simulink model "ParachuteSimV1"  (R2024b)
settings: Solver=ode5  StartTime=0.0  StopTime=1000  FixedStep=.1  RelTol=1e-3
model workspace (MAT data in the model file):
  dayOfYear = 182
  drogueArea = 1.2
  drogueCd = 2.2
  mass = 45
  rocketHorizontalArea = 3.2
  rocketHorizontalCd = 0.8
  rocketHorizontalCd1 = 0.4
  rocketMass = 165
  secOfDayUTC = 43200
  test = 1
  year = 2025
values from neighbouring files (symbols this model uses):
  apogeeHeight = ZeDeviation.*randn(numSim,1) + ZeInitial    [ParachuteSimV1.m]
  density = 0.004    [SnatchForceCalc.m]    (also in SnatchForceCalcTR.m = 1.2)
  eastwardVelocity = 30    [ParachuteSimV1.m]
  g = 9.81    [ParachuteSimV1.m]
  lattitude = 40.861903    [ParachuteSimV1.m]
  longitude = -119.113646    [ParachuteSimV1.m]
  northwardVelocity = 30    [ParachuteSimV1.m]
undefined symbols (not defined in the file or in its folder): DiscIntNeverNeededParam, Earth, WGS84, WInitialMPS
libraries: simulink x5, aerolibatmos2 x1, aerolibtransform2 x1
settings Model: PacingRate=0.100000  Creator=siyfo  LastModifiedBy=siyfo

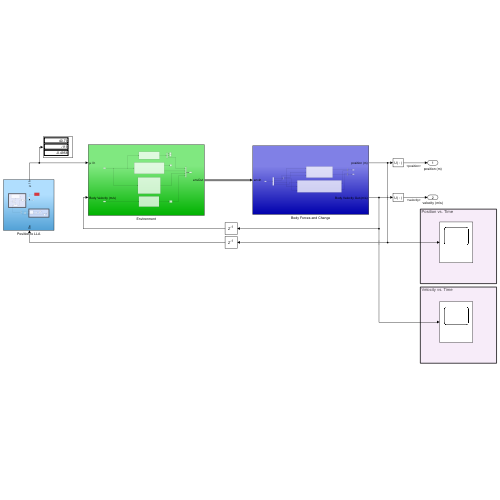
[thumbnail: Simulink's stored preview of the top-level diagram]
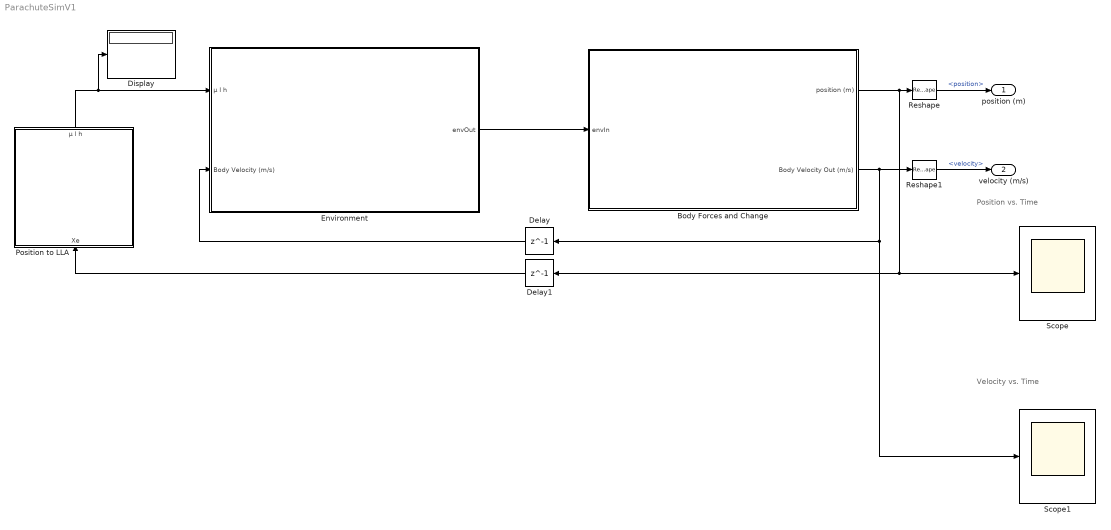
== system ParachuteSimV1 ==
  note: Position vs. Time
  note: Velocity vs. Time
  Body Forces and Change : Subsystem
  Delay : Delay  DelayLength=1  InitialCondition=0
  Delay1 : Delay  DelayLength=1  InitialCondition=0
  Display : Display
  Environment : Subsystem
  Position to LLA : Subsystem
      settings: PortSchema="{\"entries\":[{\"content\":{\"sides\":[{\"content\":{},\"type\":\"ConnectorPlacement.EquallySpacedRectSide\",\"uuid\":\"395108a1-2b9e-4f25-b149-7e7a55081f25\"},{\"content\":{\"side\":\"RIGHT\"},\"type\":\"ConnectorPlacement.EquallySpacedRectSide\",\"uuid\":\"27b5f7e2-b846-4579-8541-6937c01c751e\"},{\"content\":{\"connectorIds\":[\"Out1\"],\"side\":\"TOP\"},\"type\":\"ConnectorPlacement.EquallySpacedRectSide\",\"uuid\":\"43ca551c-6ed4-44f9-86d9-aa9f5a015e71\"},{\"content\":{\"connectorIds\":[\"In1\"],\"side\":\"BOTTOM\"},\"type\":\"ConnectorPlacement.EquallySpacedRectSide\",\"uuid\":\"6a16c409-2c2d-4a86-9d37-b69d0f58a179\"}]},\"type\":\"ConnectorPlacement.EquallySpacedConnector\",\"uuid\":\"59df7613-7675-4f40-93a5-9c85f63bdba2\"}],\"packageUris\":[\"http://schema.mathworks.com/mf0/Connector/R2020b\"],\"version\":\"1.0\"}"
  Reshape : Reshape  OutputDimensions=[1]
  Reshape1 : Reshape  OutputDimensions=[1]
  Scope : Scope
  Scope1 : Scope
  position (m) : Outport
  velocity (m/s) : Outport  Port=2  Unit=m/s
  wires:
  Environment/1(envOut) -> Body Forces and Change/1(envIn)
  Body Forces and Change/2(Body Velocity Out (m/s)) -> Reshape1/1, Delay/1, Scope1/1
  Position to LLA/1(μ l h) -> Display/1, Environment/1(μ l h)
  Delay1/1 -> Position to LLA/1(Xe)
  Delay/1 -> Environment/2(Body Velocity (m/s))
  Body Forces and Change/1(position (m)) -> Reshape/1, Scope/1, Delay1/1
  Reshape/1 -> position (m)/1  "<position>"
  Reshape1/1 -> velocity (m/s)/1  "<velocity>"

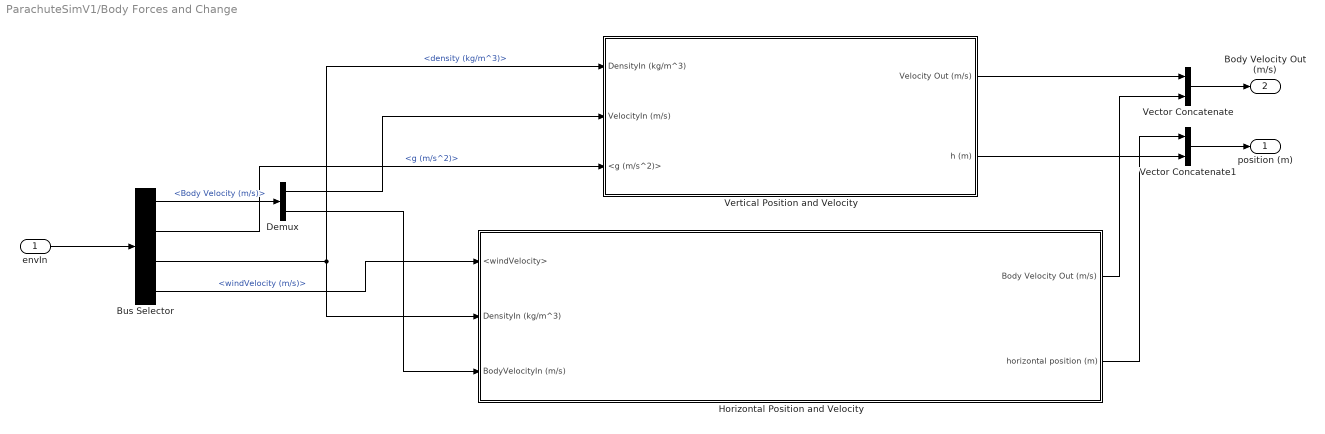
== system ParachuteSimV1/Body Forces and Change ==
  envIn : Inport
  Bus Selector : BusSelector  OutputSignals=Body Velocity (m/s),g (m/s^2),density (kg/m^3),windVelocity (m/s)
  Demux : Demux  Outputs=2
  Horizontal Position and Velocity : Subsystem
  Vector Concatenate : Concatenate  Mode=Multidimensional array
  Vector Concatenate1 : Concatenate  Mode=Multidimensional array
  Vertical Position and Velocity : Subsystem
  position (m) : Outport
  Body Velocity Out (m/s) : Outport  Port=2
  wires:
  envIn/1 -> Bus Selector/1
  Bus Selector/1 -> Demux/1  "<Body Velocity (m/s)>"
  Bus Selector/4 -> Horizontal Position and Velocity/1(<windVelocity>)  "<windVelocity (m/s)>"
  Bus Selector/3 -> Vertical Position and Velocity/1(DensityIn (kg/m^3)), Horizontal Position and Velocity/2(DensityIn (kg/m^3))  "<density (kg/m^3)>"
  Bus Selector/2 -> Vertical Position and Velocity/3(<g (m/s^2)>)  "<g (m/s^2)>"
  Vertical Position and Velocity/1(Velocity Out (m/s)) -> Vector Concatenate/1
  Demux/2 -> Horizontal Position and Velocity/3(BodyVelocityIn (m/s))
  Demux/1 -> Vertical Position and Velocity/2(VelocityIn (m/s))
  Vertical Position and Velocity/2(h (m)) -> Vector Concatenate1/2
  Vector Concatenate/1 -> Body Velocity Out (m/s)/1
  Vector Concatenate1/1 -> position (m)/1
  Horizontal Position and Velocity/2(horizontal position (m)) -> Vector Concatenate1/1
  Horizontal Position and Velocity/1(Body Velocity Out (m/s)) -> Vector Concatenate/2

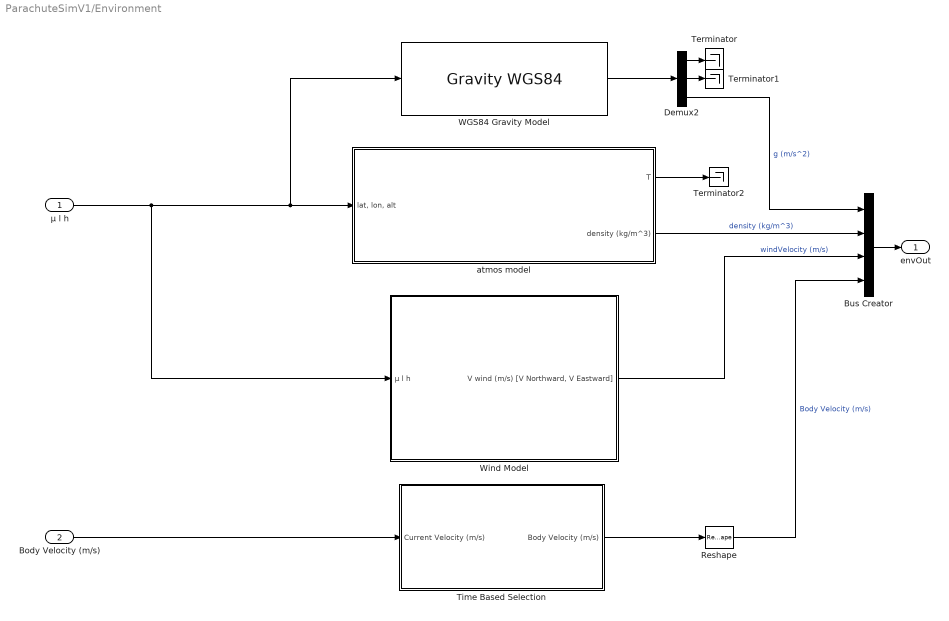
== system ParachuteSimV1/Environment ==
  μ l h : Inport
  Body Velocity (m/s) : Inport  Port=2
  Bus Creator : BusCreator  Inputs=g (m/s^2),density (kg/m^3),windVelocity (m/s),Body Velocity (m/s)
  Demux2 : Demux  Outputs=3
  Reshape : Reshape
  Terminator : Terminator
  Terminator1 : Terminator
  Terminator2 : Terminator
  Time Based Selection : Subsystem
  "WGS84 Gravity Model  " : GravityWGS84
  Wind Model : Subsystem
  atmos model : Subsystem
  envOut : Outport
  wires:
  atmos model/1(T) -> Terminator2/1
  Demux2/1 -> Terminator/1
  Demux2/2 -> Terminator1/1
  Demux2/3 -> Bus Creator/1  "g (m/s^2)"
  "WGS84 Gravity Model  "/1 -> Demux2/1
  atmos model/2(density (kg/m^3)) -> Bus Creator/2  "density (kg/m^3)"
  μ l h/1 -> atmos model/1("lat, lon, alt"), "WGS84 Gravity Model  "/1, Wind Model/1(μ l h)
  Wind Model/1("V wind (m/s) [V Northward, V Eastward]") -> Bus Creator/3  "windVelocity (m/s)"
  Bus Creator/1 -> envOut/1
  Body Velocity (m/s)/1 -> Time Based Selection/1(Current Velocity (m/s))
  Time Based Selection/1(Body Velocity (m/s)) -> Reshape/1
  Reshape/1 -> Bus Creator/4  "Body Velocity (m/s)"

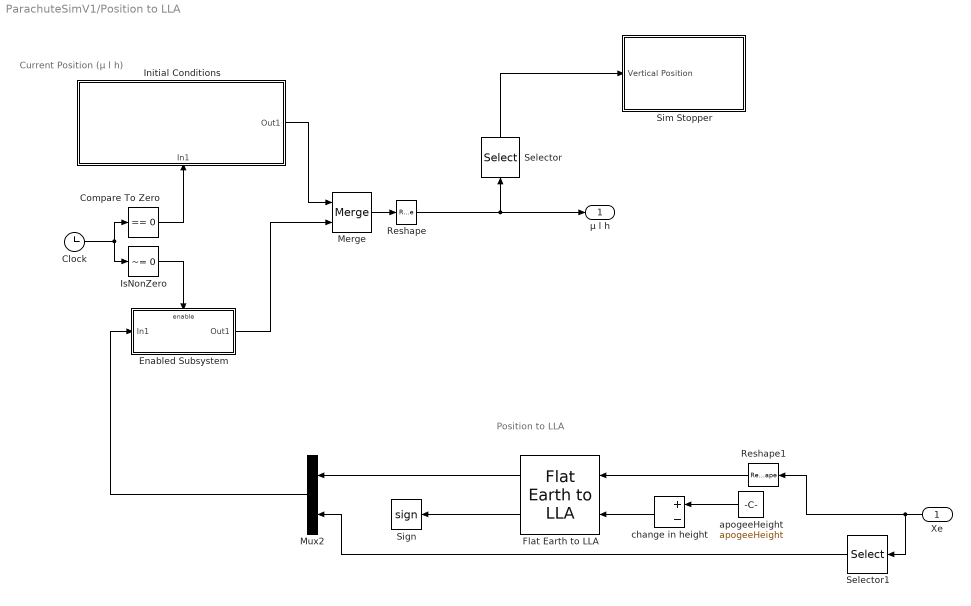
== system ParachuteSimV1/Position to LLA ==
  note: Position to LLA
  note: Current Position (μ l h)
  Xe : Inport
  Clock : Clock
  Compare To Zero : simulink/Logic and Bit Operations/Compare To Zero  relop===  OutDataTypeStr=uint8
  Enabled Subsystem : Subsystem  TreatAsAtomicUnit=on
  Flat Earth to LLA : aerolibtransform2/Flat Earth to LLA  units=Metric (MKS)  ptype=Earth (WGS84)  F=1/298.257223563  R=6378137  refPosPort=off  LL0=[lattitude longitude]  psi=90
  Initial Conditions : Subsystem
      settings: PortSchema="{\"entries\":[{\"content\":{\"sides\":[{\"content\":{},\"type\":\"ConnectorPlacement.EquallySpacedRectSide\",\"uuid\":\"693e8934-6ee4-461b-8cf6-42b2b2261af3\"},{\"content\":{\"connectorIds\":[\"Out1\"],\"side\":\"RIGHT\"},\"type\":\"ConnectorPlacement.EquallySpacedRectSide\",\"uuid\":\"27a2a18d-addc-401c-ab89-c55f8d21a6b0\"},{\"content\":{\"side\":\"TOP\"},\"type\":\"ConnectorPlacement.EquallySpacedRectSide\",\"uuid\":\"aace6f03-20fd-4ea0-8b41-e6402498191a\"},{\"content\":{\"connectorIds\":[\"In1\"],\"side\":\"BOTTOM\"},\"type\":\"ConnectorPlacement.EquallySpacedRectSide\",\"uuid\":\"e2c8b452-2239-4d25-8a3f-abbb82eaafca\"}]},\"type\":\"ConnectorPlacement.EquallySpacedConnector\",\"uuid\":\"08404bb2-7ad5-42d3-9682-7974a009b565\"}],\"packageUris\":[\"http://schema.mathworks.com/mf0/Connector/R2020b\"],\"version\":\"1.0\"}"
  IsNonZero : simulink/Logic and Bit Operations/Compare To Zero  relop=~=  OutDataTypeStr=boolean
      settings: LibrarySourceBlock=|
      | simulink/Quick Insert/Logic and Bit
      | Operations/IsNonZero
  Merge : Merge
  Mux2 : Mux  Inputs=2
  Reshape : Reshape
  Reshape1 : Reshape
  Selector : Selector  InputPortWidth=3  IndexOptions=Index vector (dialog)  Indices=[3]  OutputSizes=1
  Selector1 : Selector  InputPortWidth=3  IndexOptions=Index vector (dialog)  Indices=[3]  OutputSizes=1
  Sign : Signum
  Sim Stopper : Subsystem
  apogeeHeight : Constant  Value=apogeeHeight
  change in height : Sum  Inputs=+-
  μ l h : Outport
  wires:
  IsNonZero/1 -> Enabled Subsystem/Enable
  Compare To Zero/1 -> Initial Conditions/1(In1)
  Initial Conditions/1(Out1) -> Merge/1
  Enabled Subsystem/1(Out1) -> Merge/2
  Flat Earth to LLA/1 -> Mux2/1
  Clock/1 -> Compare To Zero/1, IsNonZero/1
  Merge/1 -> Reshape/1
  Xe/1 -> Reshape1/1, Selector1/1
  Flat Earth to LLA/2 -> Sign/1
  Selector1/1 -> Mux2/2
  apogeeHeight/1 -> change in height/1
  change in height/1 -> Flat Earth to LLA/2
  Reshape1/1 -> Flat Earth to LLA/1
  Mux2/1 -> Enabled Subsystem/1(In1)
  Selector/1 -> Sim Stopper/1(Vertical Position)
  Reshape/1 -> Selector/1, μ l h/1

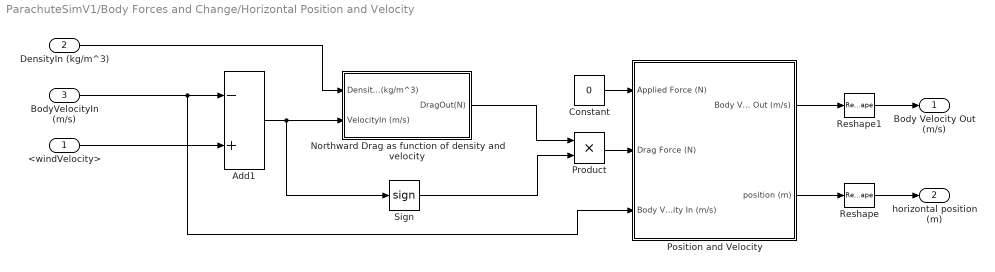
== system ParachuteSimV1/Body Forces and Change/Horizontal Position and Velocity ==
  <windVelocity> : Inport
  DensityIn (kg/m^3) : Inport  Port=2
  BodyVelocityIn (m/s) : Inport  Port=3
  Add1 : Sum  Inputs=-+
  Constant : Constant  Value=0
  Northward Drag as function of density and velocity : Subsystem
  Position and Velocity : Subsystem
  Product : Product
  Reshape : Reshape
  Reshape1 : Reshape
  Sign : Signum
  Body Velocity Out (m/s) : Outport
  horizontal position (m) : Outport  Port=2  OutDataTypeStr=fixdt('double', 'DataTypeOverride', 'Off')
  wires:
  <windVelocity>/1 -> Add1/2
  Constant/1 -> Position and Velocity/1(Applied Force (N))
  Sign/1 -> Product/2
  DensityIn (kg/m^3)/1 -> Northward Drag as function of density and velocity/1(DensityIn (kg/m^3))
  Position and Velocity/2(position (m)) -> Reshape/1
  Add1/1 -> Sign/1, Northward Drag as function of density and velocity/2(VelocityIn (m/s))
  Position and Velocity/1(Body Velocity Out (m/s)) -> Reshape1/1
  BodyVelocityIn (m/s)/1 -> Position and Velocity/3(Body Velocity In (m/s)), Add1/1
  Reshape/1 -> horizontal position (m)/1
  Reshape1/1 -> Body Velocity Out (m/s)/1
  Northward Drag as function of density and velocity/1(DragOut(N)) -> Product/1
  Product/1 -> Position and Velocity/2(Drag Force (N))

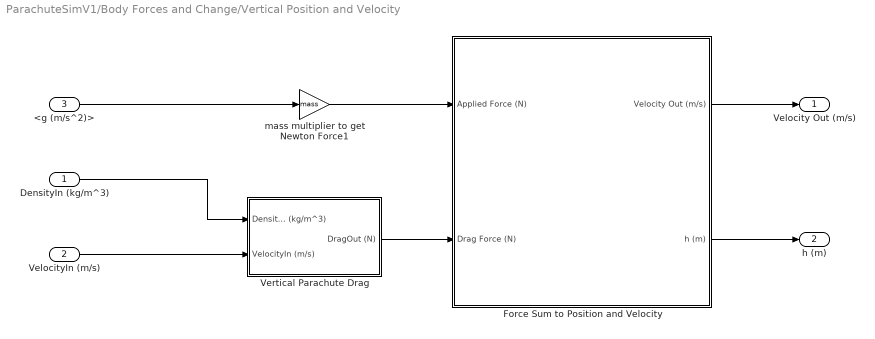
== system ParachuteSimV1/Body Forces and Change/Vertical Position and Velocity ==
  DensityIn (kg/m^3) : Inport
  VelocityIn (m/s) : Inport  Port=2
  <g (m/s^2)> : Inport  Port=3
  Force Sum to Position and Velocity : Subsystem
  Vertical Parachute Drag : Subsystem
  mass multiplier to get Newton Force1 : Gain  Gain=mass
  Velocity Out (m/s) : Outport
  h (m) : Outport  Port=2
  wires:
  Vertical Parachute Drag/1(DragOut (N)) -> Force Sum to Position and Velocity/2(Drag Force (N))
  DensityIn (kg/m^3)/1 -> Vertical Parachute Drag/1(DensityIn (kg/m^3))
  VelocityIn (m/s)/1 -> Vertical Parachute Drag/2(VelocityIn (m/s))
  mass multiplier to get Newton Force1/1 -> Force Sum to Position and Velocity/1(Applied Force (N))
  <g (m/s^2)>/1 -> mass multiplier to get Newton Force1/1
  Force Sum to Position and Velocity/2(h (m)) -> h (m)/1
  Force Sum to Position and Velocity/1(Velocity Out (m/s)) -> Velocity Out (m/s)/1

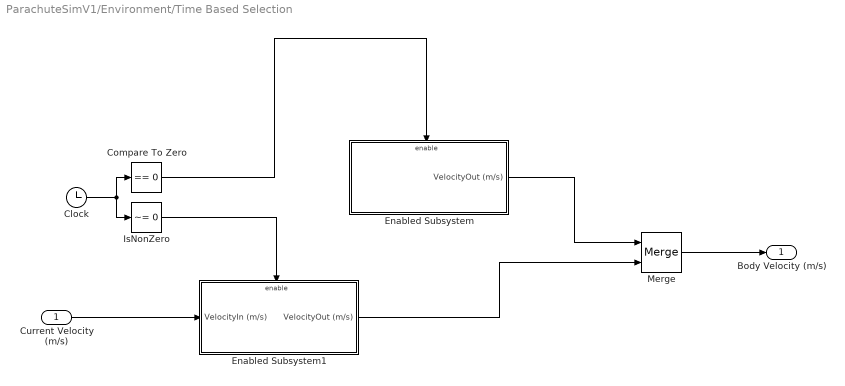
== system ParachuteSimV1/Environment/Time Based Selection ==
  Current Velocity (m/s) : Inport
  Clock : Clock
  Compare To Zero : simulink/Logic and Bit Operations/Compare To Zero  relop===  OutDataTypeStr=uint8
  Enabled Subsystem : Subsystem  TreatAsAtomicUnit=on
  Enabled Subsystem1 : Subsystem  TreatAsAtomicUnit=on
  IsNonZero : simulink/Logic and Bit Operations/Compare To Zero  relop=~=  OutDataTypeStr=boolean
  Merge : Merge
  Body Velocity (m/s) : Outport
  wires:
  Current Velocity (m/s)/1 -> Enabled Subsystem1/1(VelocityIn (m/s))
  Clock/1 -> Compare To Zero/1, IsNonZero/1
  IsNonZero/1 -> Enabled Subsystem1/Enable
  Compare To Zero/1 -> Enabled Subsystem/Enable
  Enabled Subsystem1/1(VelocityOut (m/s)) -> Merge/2
  Enabled Subsystem/1(VelocityOut (m/s)) -> Merge/1
  Merge/1 -> Body Velocity (m/s)/1

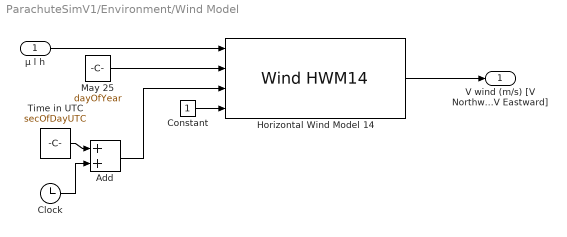
== system ParachuteSimV1/Environment/Wind Model ==
  μ l h : Inport
  Add : Sum
  Clock : Clock
  Constant : Constant
  Horizontal Wind Model 14 : WindHWM14  model=Total  action=Warning
  May 25 : Constant  Value=dayOfYear
  Time in UTC : Constant  Value=secOfDayUTC
  "V wind (m/s) [V Northward, V Eastward]" : Outport
  wires:
  May 25/1 -> Horizontal Wind Model 14/2
  Add/1 -> Horizontal Wind Model 14/3
  Time in UTC/1 -> Add/1
  Constant/1 -> Horizontal Wind Model 14/4
  Clock/1 -> Add/2
  μ l h/1 -> Horizontal Wind Model 14/1
  Horizontal Wind Model 14/1 -> "V wind (m/s) [V Northward, V Eastward]"/1

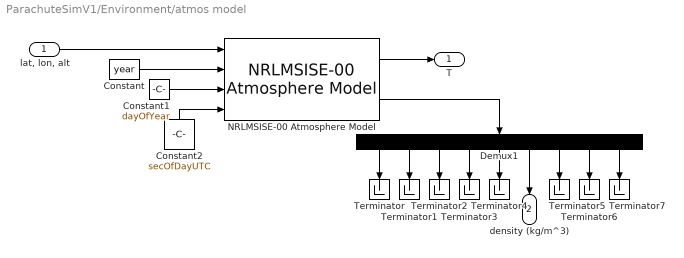
== system ParachuteSimV1/Environment/atmos model ==
  "lat, lon, alt" : Inport
  Constant : Constant  Value=year
  Constant1 : Constant  Value=dayOfYear
  Constant2 : Constant  Value=secOfDayUTC
  Demux1 : Demux  Outputs=9
  NRLMSISE-00 Atmosphere Model : aerolibatmos2/NRLMSISE-00 Atmosphere Model  units=Metric (MKS)  lst_input=off  flux_ap_input=off  flags_input=Internal  flags=ones(1,23)  oxygen_in=off  action=Warning
  Terminator{,1..7} (8 alike) : Terminator
  T : Outport
  density (kg/m^3) : Outport  Port=2  OutDataTypeStr=double
  wires:
  Demux1/6 -> density (kg/m^3)/1
  "lat, lon, alt"/1 -> NRLMSISE-00 Atmosphere Model/1
  NRLMSISE-00 Atmosphere Model/2 -> Demux1/1
  Constant1/1 -> NRLMSISE-00 Atmosphere Model/3
  Constant/1 -> NRLMSISE-00 Atmosphere Model/2
  Constant2/1 -> NRLMSISE-00 Atmosphere Model/4
  NRLMSISE-00 Atmosphere Model/1 -> T/1
  Demux1/1 -> Terminator/1
  Demux1/7 -> Terminator5/1
  Demux1/8 -> Terminator6/1
  Demux1/9 -> Terminator7/1
  Demux1/5 -> Terminator4/1
  Demux1/4 -> Terminator3/1
  Demux1/3 -> Terminator2/1
  Demux1/2 -> Terminator1/1

== system ParachuteSimV1/Position to LLA/Enabled Subsystem ==
  In1 : Inport
  Enable : EnablePort
  Out1 : Outport
  wires:
  In1/1 -> Out1/1

== system ParachuteSimV1/Position to LLA/Initial Conditions ==
  In1 : Inport
  Enabled Subsystem : Subsystem  TreatAsAtomicUnit=on
  Mux : Mux  Inputs=3
  height : Constant  Value=apogeeHeight
  lat : Constant  Value=lattitude
  long : Constant  Value=longitude
  Out1 : Outport
  wires:
  long/1 -> Mux/2
  In1/1 -> Enabled Subsystem/Enable
  Mux/1 -> Enabled Subsystem/1(In1)
  Enabled Subsystem/1(Out1) -> Out1/1
  lat/1 -> Mux/1
  height/1 -> Mux/3

== system ParachuteSimV1/Position to LLA/Sim Stopper ==
  Vertical Position : Inport
  Constant : Constant
  Enabled Subsystem1 : Subsystem  TreatAsAtomicUnit=on
  IsZero : simulink/Logic and Bit Operations/Compare To Zero  relop=<=  OutDataTypeStr=boolean
  Stop Simulation : Stop
  wires:
  Vertical Position/1 -> IsZero/1
  Enabled Subsystem1/1(Out1) -> Stop Simulation/1
  Constant/1 -> Enabled Subsystem1/1(In1)
  IsZero/1 -> Enabled Subsystem1/Enable

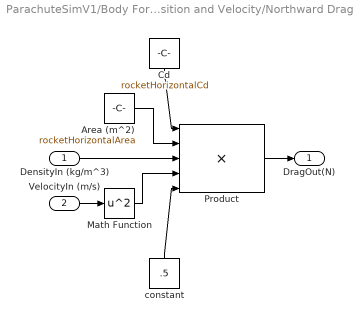
== system ParachuteSimV1/Body Forces and Change/Horizontal Position and Velocity/Northward Drag as function of density and velocity ==
  DensityIn (kg/m^3) : Inport
  VelocityIn (m/s) : Inport  Port=2
  Area (m^2) : Constant  Value=rocketHorizontalArea
  Cd : Constant  Value=rocketHorizontalCd
  Math Function : Math  Operator=square
  Product : Product  Inputs=5
  constant : Constant  Value=.5
  DragOut(N) : Outport
  wires:
  Cd/1 -> Product/1
  Area (m^2)/1 -> Product/2
  DensityIn (kg/m^3)/1 -> Product/3
  constant/1 -> Product/5
  Product/1 -> DragOut(N)/1
  VelocityIn (m/s)/1 -> Math Function/1
  Math Function/1 -> Product/4

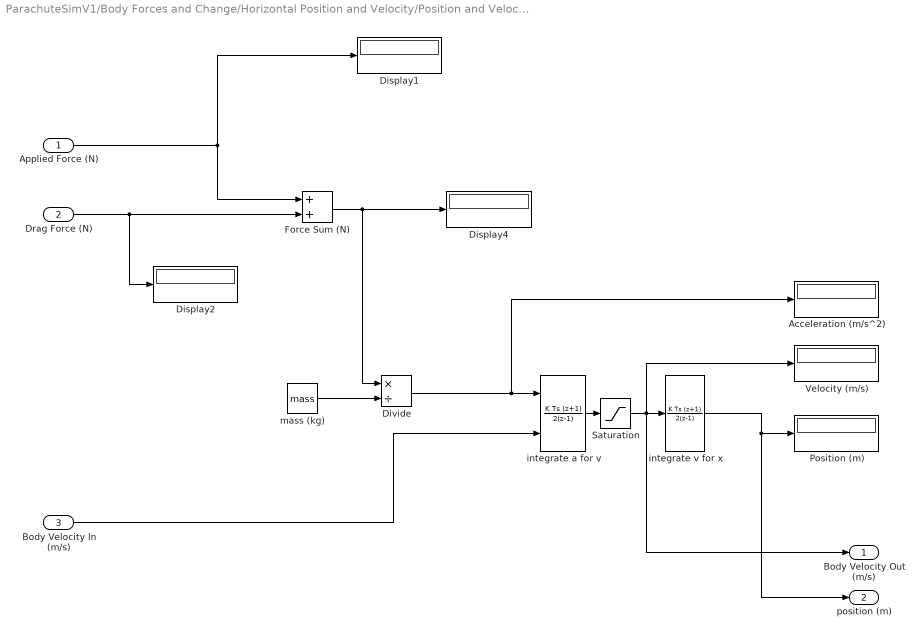
== system ParachuteSimV1/Body Forces and Change/Horizontal Position and Velocity/Position and Velocity ==
  Applied Force (N) : Inport
  Drag Force (N) : Inport  Port=2
  Body Velocity In (m/s) : Inport  Port=3
  Acceleration (m/s^2) : Display
      settings: Format=bank
  Display1 : Display
      settings: Format=bank
  Display2 : Display
      settings: Format=bank
  Display4 : Display
      settings: Format=bank
  Divide : Product  Inputs=*/  OutDataTypeStr=double
  Force Sum (N) : Sum
  Position (m) : Display
      settings: Format=bank
  Saturation : Saturate  UpperLimit=150  LowerLimit=-150
  Velocity (m/s) : Display
      settings: Format=bank
  integrate a for v : DiscreteIntegrator  IntegratorMethod=Integration: Trapezoidal  InitialConditionSource=external  InitialCondition=northwardVelocity  SampleTime=-1  OutMin=[-300]  OutMax=[300]  ICPrevOutput=DiscIntNeverNeededParam  ICPrevScaledInput=DiscIntNeverNeededParam
  integrate v for x : DiscreteIntegrator  IntegratorMethod=Integration: Trapezoidal  SampleTime=-1  ICPrevOutput=DiscIntNeverNeededParam  ICPrevScaledInput=DiscIntNeverNeededParam
  mass (kg) : Constant  Value=mass
  Body Velocity Out (m/s) : Outport
  position (m) : Outport  Port=2  OutDataTypeStr=double  Unit=m  LockScale=on
  wires:
  mass (kg)/1 -> Divide/2
  Force Sum (N)/1 -> Divide/1, Display4/1
  integrate v for x/1 -> position (m)/1, Position (m)/1
  Drag Force (N)/1 -> Force Sum (N)/2, Display2/1
  Applied Force (N)/1 -> Display1/1, Force Sum (N)/1
  integrate a for v/1 -> Saturation/1
  Body Velocity In (m/s)/1 -> integrate a for v/2
  Divide/1 -> Acceleration (m/s^2)/1, integrate a for v/1
  Saturation/1 -> Velocity (m/s)/1, Body Velocity Out (m/s)/1, integrate v for x/1

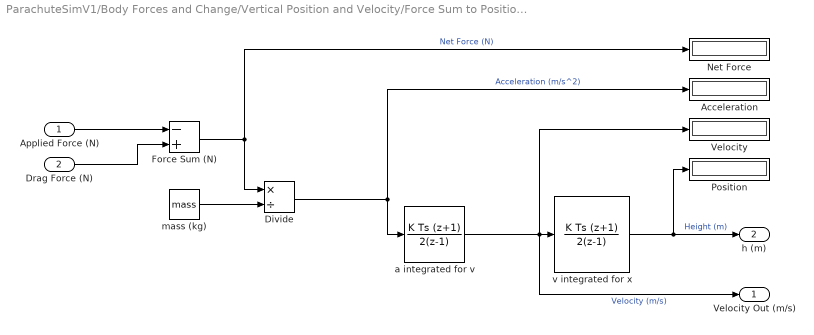
== system ParachuteSimV1/Body Forces and Change/Vertical Position and Velocity/Force Sum to Position and Velocity ==
  Applied Force (N) : Inport
  Drag Force (N) : Inport  Port=2  OutDataTypeStr=double
  Acceleration : Display
      settings: Format=bank
  Divide : Product  Inputs=*/  OutDataTypeStr=Inherit: Inherit via back propagation
  Force Sum (N) : Sum  Inputs=-+  OutDataTypeStr=double
  Net Force : Display
      settings: Format=bank
  Position : Display
      settings: Format=bank
  Velocity : Display
      settings: Format=bank
  a integrated for v : DiscreteIntegrator  IntegratorMethod=Integration: Trapezoidal  gainval=1  SampleTime=-1  ICPrevOutput=DiscIntNeverNeededParam  ICPrevScaledInput=DiscIntNeverNeededParam
  mass (kg) : Constant  Value=mass
  v integrated for x : DiscreteIntegrator  IntegratorMethod=Integration: Trapezoidal  InitialCondition=apogeeHeight  SampleTime=-1  ICPrevOutput=DiscIntNeverNeededParam  ICPrevScaledInput=DiscIntNeverNeededParam
  Velocity Out (m/s) : Outport  OutDataTypeStr=double
  h (m) : Outport  Port=2
  wires:
  mass (kg)/1 -> Divide/2
  Force Sum (N)/1 -> Net Force/1, Divide/1  "Net Force (N)"
  v integrated for x/1 -> Position/1, h (m)/1  "Height (m)"
  Drag Force (N)/1 -> Force Sum (N)/2
  Applied Force (N)/1 -> Force Sum (N)/1
  a integrated for v/1 -> Velocity/1, Velocity Out (m/s)/1, v integrated for x/1  "Velocity (m/s)"
  Divide/1 -> Acceleration/1, a integrated for v/1  "Acceleration (m/s^2)"

== system ParachuteSimV1/Body Forces and Change/Vertical Position and Velocity/Vertical Parachute Drag ==
  DensityIn (kg/m^3) : Inport
  VelocityIn (m/s) : Inport  Port=2
  (m^2/s^2) : Math  Operator=square
  Area (m^2) : Constant  Value=drogueArea
  Cd : Constant  Value=drogueCd
  Product : Product  Inputs=5  OutDataTypeStr=double
  constant : Constant  Value=.5
  DragOut (N) : Outport  OutDataTypeStr=double
  wires:
  Area (m^2)/1 -> Product/2
  DensityIn (kg/m^3)/1 -> Product/3
  constant/1 -> Product/5
  Product/1 -> DragOut (N)/1
  VelocityIn (m/s)/1 -> (m^2/s^2)/1
  (m^2/s^2)/1 -> Product/4
  Cd/1 -> Product/1

== system ParachuteSimV1/Environment/Time Based Selection/Enabled Subsystem ==
  Enable : EnablePort
  Mux : Mux  Inputs=3
  eastwardVelocity (m/s) : Constant  Value=eastwardVelocity
  northwardVelocity (m/s) : Constant  Value=northwardVelocity
  verticalVelocity (m/s) : Constant  Value=WInitialMPS
  VelocityOut (m/s) : Outport
  wires:
  northwardVelocity (m/s)/1 -> Mux/2
  eastwardVelocity (m/s)/1 -> Mux/3
  Mux/1 -> VelocityOut (m/s)/1
  verticalVelocity (m/s)/1 -> Mux/1

== system ParachuteSimV1/Environment/Time Based Selection/Enabled Subsystem1 ==
  VelocityIn (m/s) : Inport
  Enable : EnablePort
  VelocityOut (m/s) : Outport
  wires:
  VelocityIn (m/s)/1 -> VelocityOut (m/s)/1

== system ParachuteSimV1/Position to LLA/Initial Conditions/Enabled Subsystem ==
  In1 : Inport
  Enable : EnablePort
  Out1 : Outport
  wires:
  In1/1 -> Out1/1

== system ParachuteSimV1/Position to LLA/Sim Stopper/Enabled Subsystem1 ==
  In1 : Inport
  Enable : EnablePort
  Out1 : Outport
  wires:
  In1/1 -> Out1/1
